simulink library "libraries"  (R2016b)
settings: Solver=VariableStepAuto  StartTime=0.0  StopTime=10.0  RelTol=1e-3
values from neighbouring files (symbols this model uses):
  MIN_SAFE_DIST = 1    [simulation.m]    (also in stateflowSim.m)
  WORLD_SIZE = 8    [simulation.m]    (also in stateflowSim.m)
undefined symbols (not defined in the file or in its folder): dt, V_MIN, V_TURN
settings Model: Creator=larry  LastModifiedBy=larry

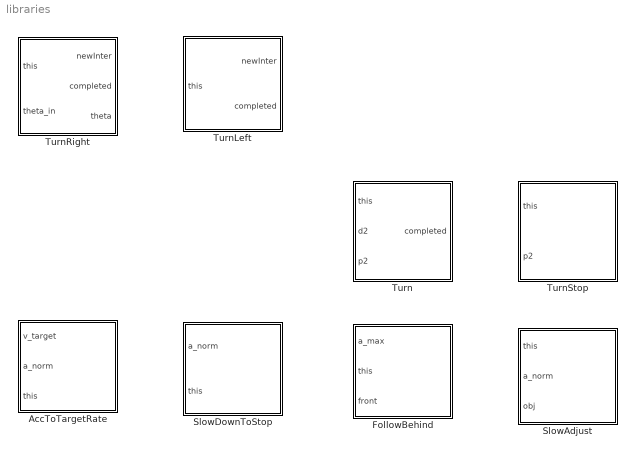
== system libraries ==
  AccToTargetRate : Stateflow chart  TreatAsAtomicUnit=on
  FollowBehind : Stateflow chart  TreatAsAtomicUnit=on
  SlowAdjust : Stateflow chart  TreatAsAtomicUnit=on
  SlowDownToStop : Stateflow chart  TreatAsAtomicUnit=on
  Turn : Stateflow chart  TreatAsAtomicUnit=on
  TurnLeft : Stateflow chart  TreatAsAtomicUnit=on
  TurnRight : Stateflow chart  TreatAsAtomicUnit=on
  TurnStop : Stateflow chart  TreatAsAtomicUnit=on

== stateflow chart libraries/AccToTargetRate ==
  state AccFromStop
    en:
    a = D(:,this) * a_norm;
    du:
    accelerate(this);
  state FixRate
    en:
    a = D(:,this) * 0;
    du:
    fixedRateDrive(this);
  (default) -> AccFromStop [order 2]
  AccFromStop -> FixRate : [reachTargetRate(this)]
  (default) -> FixRate [order 1] : [reachTargetRate(this)]
  data: self function_input uint8 size=1; self function_input uint8 size=1; self function_input uint8 size=1; res function_output boolean size=1; V data_store_memory; D data_store_memory; v_target input double size=1; a_norm input double size=1; this input uint8 size=1 =uint8(1); WORLD_SIZE parameter; a local double size=[2 1]; dt parameter; X data_store_memory
  function fixedRateDrive(self):
    | function fixedRateDrive(self)
    |  
    | x = X(:,self);
    | v = V(:,self);
    | 
    | % update new position
    | x = x + v * dt;
    | 
    | % a rounded world
    | if x(1) > WORLD_SIZE
    |     x(1) = -WORLD_SIZE;
    | elseif x(1) < -WORLD_SIZE
    |     x(1) = WORLD_SIZE;
    | elseif x(2) > WORLD_SIZE
    |     x(2) = -WORLD_SIZE;
    | elseif x(2) < -WORLD_SIZE
    |     x(2) = WORLD_SIZE;
    | end
    | 
    | X(:,self) = x;
  function accelerate(self):
    | function accelerate(self)
    | 
    | x = X(:,self);
    | v = V(:,self);
    | 
    | x = x + v * dt + 0.5 * a * dt * dt;
    | v = v + a * dt;
    | 
    | % a rounded world
    | if x(1) > WORLD_SIZE
    |     x(1) = -WORLD_SIZE;
    | elseif x(1) < -WORLD_SIZE
    |     x(1) = WORLD_SIZE;
    | elseif x(2) > WORLD_SIZE
    |     x(2) = -WORLD_SIZE;
    | elseif x(2) < -WORLD_SIZE
    |     x(2) = WORLD_SIZE;
    | end
    | 
    | X(:,self) = x;
    | V(:,self) = v;
  function res = reachTargetRate(self):
    | function res = reachTargetRate(self)
    | 
    | res = (norm(V(:,self)) >= v_target);

== stateflow chart libraries/SlowDownToStop ==
  state SlowToStop
    en:
    a = (-1) * D(:,this) * a_norm;
    du:
    accelerate(this);
  state Stop
    en:
    a = D(:,this) * 0;
    V(:,this) = V(:,this) * 0;
  (default) -> SlowToStop [order 2]
  SlowToStop -> Stop : [isStopped(this)]
  (default) -> Stop [order 1] : [isStopped(this)]
  data: self function_input uint8 size=1; self function_input uint8 size=1; res function_output boolean size=1; V data_store_memory; D data_store_memory; a_norm input double size=1; this input uint8 size=1 =uint8(1); WORLD_SIZE parameter; a local double size=[2 1]; dt parameter; X data_store_memory; V_MIN parameter
  function accelerate(self):
    | function accelerate(self)
    | 
    | x = X(:,self);
    | v = V(:,self);
    | 
    | x = x + v * dt + 0.5 * a * dt * dt;
    | v = v + a * dt;
    | 
    | % a rounded world
    | if x(1) > WORLD_SIZE
    |     x(1) = -WORLD_SIZE;
    | elseif x(1) < -WORLD_SIZE
    |     x(1) = WORLD_SIZE;
    | elseif x(2) > WORLD_SIZE
    |     x(2) = -WORLD_SIZE;
    | elseif x(2) < -WORLD_SIZE
    |     x(2) = WORLD_SIZE;
    | end
    | 
    | X(:,self) = x;
    | V(:,self) = v;
  function res = isStopped(self):
    | function res = isStopped(self)
    | 
    | v = V(:,self);
    | d = D(:,self);
    | res = (dot(v, d) <= 0)||(norm(v) < V_MIN);

== stateflow chart libraries/FollowBehind ==
  state Follow
    du:
    followFrontCar(this,front)
  (default) -> Follow
  data: self function_input uint8 size=1; index function_input uint8 size=1; V data_store_memory; D data_store_memory; a_max input double size=1; this input uint8 size=1 =uint8(1); WORLD_SIZE parameter; dt parameter; X data_store_memory; front input; MIN_SAFE_DIST parameter
  function followFrontCar(self, index):
    | function followFrontCar(self, index)
    | 
    | x = X(:,self);
    | v = V(:,self);
    | d = D(:,self);
    | a = [0; 0];
    | 
    | xfront = X(:,index);
    | vfront = V(:,index);
    | 
    | range = 2 * WORLD_SIZE;
    | dist = mod((dot(xfront - x, d)+range), range);
    | 
    | v_norm = norm(v);
    | vfront_norm = dot(vfront, d);
    | 
    | if dist <= 2*MIN_SAFE_DIST 
    |     
    |     if v_norm >= vfront_norm 
    |         vo = d * vfront_norm;
    |         if dist <= 1.5*MIN_SAFE_DIST
    |             vo = 0.75*vo;
    |         elseif dist <= MIN_SAFE_DIST
    |             vo = 0.5*vo;
    |         end
    |     else
    |         if dist <= MIN_SAFE_DIST
    |             vo = d * (v_norm + (vfront_norm - v_norm)*0.2);
    |         else
    |             vo = d * (v_norm + (vfront_norm - v_norm)*0.4);
    |         end
    |     end
    |     
    |     ar = (vo - v) / dt;
    |     ar_norm = norm(ar);
    |     if ar_norm > a_max
    |         ar = ar/ar_norm * a_max;
    |         x = x + v * dt + 0.5 * ar * dt * dt;
    |         v = v + ar * dt;
    |     else
    |         x = x + (v + vo) * dt / 2;
    |         v = vo;
    |     end
    |     a = ar;
    | else
    |     x = x + v * dt;
    | end
    | 
    | % a rounded world
    | if x(1) > WORLD_SIZE
    |     x(1) = -WORLD_SIZE;
    | elseif x(1) < -WORLD_SIZE
    |     x(1) = WORLD_SIZE;
    | elseif x(2) > WORLD_SIZE
    |     x(2) = -WORLD_SIZE;
    | elseif x(2) < -WORLD_SIZE
    |     x(2) = WORLD_SIZE;
    | end
    | 
    | X(:,self) = x;
    | V(:,self) = v;

== stateflow chart libraries/SlowAdjust ==
  state SlowDown
    en:
    a = (-1) * D(:,this) * a_norm;
    du:
    accelerate(this);
  state Adjust
    du:
    adjustBehind(this,obj)
  (default) -> SlowDown [order 2]
  SlowDown -> Adjust : [isStopped(this)]
  (default) -> Adjust [order 1] : [isStopped(this)]
  data: self function_input uint8 size=1; self function_input uint8 size=1; res function_output boolean size=1; self function_input uint8 size=1; pos function_input double size=[2 1]; V data_store_memory; D data_store_memory; this input uint8 size=1 =uint8(1); WORLD_SIZE parameter; dt parameter; X data_store_memory; MIN_SAFE_DIST parameter; V_MIN parameter; a local; a_norm input double size=1; obj input double size=[2 1]
  function accelerate(self):
    | function accelerate(self)
    | 
    | x = X(:,self);
    | v = V(:,self);
    | 
    | x = x + v * dt + 0.5 * a * dt * dt;
    | v = v + a * dt;
    | 
    | % a rounded world
    | if x(1) > WORLD_SIZE
    |     x(1) = -WORLD_SIZE;
    | elseif x(1) < -WORLD_SIZE
    |     x(1) = WORLD_SIZE;
    | elseif x(2) > WORLD_SIZE
    |     x(2) = -WORLD_SIZE;
    | elseif x(2) < -WORLD_SIZE
    |     x(2) = WORLD_SIZE;
    | end
    | 
    | X(:,self) = x;
    | V(:,self) = v;
  function res = isStopped(self):
    | function res = isStopped(self)
    | 
    | v = V(:,self);
    | d = D(:,self);
    | res = (dot(v, d) <= 0)||(norm(v) < V_MIN);
  function adjustBehind(self,pos):
    | function adjustBehind(self,pos)
    | 
    | x = X(:,self);
    | v = V(:,self);
    | d = D(:,self);
    | 
    | assert(norm(v) <= V_MIN);
    | 
    | diff = dot(pos - x, d);
    | if diff > MIN_SAFE_DIST
    |     v = V_MIN * d;
    |     dx_norm = V_MIN * dt;
    |     if (diff - dx_norm) >= MIN_SAFE_DIST
    |         x = x + dx_norm * d;
    |     else
    |         x = pos - MIN_SAFE_DIST * d;
    |     end
    | else
    |     v = 0 * v;
    | end
    | 
    | X(:,self) = x;
    | V(:,self) = v;

== stateflow chart libraries/TurnRight ==
  state Turn
    en:
    prepareRightTurn(this);
    check = false;
    du:
    check = rightTurn(this);
  state Resume
    en:
    newInter = ...
    resumeFromRightTurn(this);
    completed = true;
  (default) -> Turn
  Turn -> Resume : [check]
  data: self function_input uint8 size=1; self function_input uint8 size=1; res function_output boolean size=1; self function_input uint8 size=1; inter function_output double size=[2 1]; V data_store_memory; D data_store_memory; this input uint8 size=1 =uint8(1); dt parameter; X data_store_memory; dth local double size=1 =10; p0 local; x0 local; d0 local; newInter output; check local; completed output; vturn local; theta_in input; theta output double size=1 =0
  function prepareRightTurn(self):
    | function prepareRightTurn(self)
    | 
    | r = 0.5;
    | d0 = D(:,self);
    | theta = theta_in;
    | vturn = r * deg2rad(dth) / dt;
    | 
    | if isequal(d0, [1; 0])
    |     x0 = [-1; -0.5];
    |     p0 = [0; 0.5];
    | elseif isequal(d0, [-1; 0])
    |     x0 = [1; 0.5];
    |     p0 = [0; -0.5];
    | elseif isequal(d0, [0; 1])
    |     x0 = [0.5; -1];
    |     p0 = [-0.5; 0];
    | elseif isequal(d0, [0; -1])
    |     x0 = [-0.5; 1];
    |     p0 = [0.5; 0];
    | else
    |     error('Unknown orientation');
    | end
  function res = rightTurn(self):
    | function res = rightTurn(self)
    | 
    | res = false;
    | theta = theta + dth;
    | rad = deg2rad(theta);
    | 
    | rot = [cos(rad) sin(rad); -sin(rad) cos(rad)];
    | pf = rot * p0;
    | df = rot * d0;
    | 
    | diff = pf - p0;
    | 
    | % update states
    | X(:,self) = x0 + diff;
    | V(:,self) = df * vturn;
    | D(:,self) = df;
    | 
    | res = theta >= 90;
  function inter = resumeFromRightTurn(self):
    | function inter = resumeFromRightTurn(self)
    | 
    | if isequal(d0, [1; 0])
    |     df = [0; -1];
    |     xf = [-0.5; -1];
    |     inter = [-0.5; 1];
    | elseif isequal(d0, [-1; 0])
    |     df = [0; 1];
    |     xf = [0.5; 1];
    |     inter = [-0.5; -1];
    | elseif isequal(d0, [0; 1])
    |     df = [1; 0];
    |     xf = [1; -0.5];
    |     inter = [-1; -0.5];
    | elseif isequal(d0, [0; -1])
    |     df = [-1; 0];
    |     xf = [-1; 0.5];
    |     inter = [1; 0.5];
    | else
    |     error('Unknown orientation');
    | end
    | 
    | X(:,self) = xf;
    | V(:,self) = df * vturn;
    | D(:,self) = df;

== stateflow chart libraries/TurnLeft ==
  state Turn
    en:
    prepareLeftTurn(this);
    check = false;
    du:
    check = leftTurn(this);
  state Resume
    en:
    newInter = ...
    resumeFromLeftTurn(this);
    completed = true;
  (default) -> Turn
  Turn -> Resume : [check]
  data: self function_input uint8 size=1; self function_input uint8 size=1; res function_output boolean size=1; self function_input uint8 size=1; inter function_output double size=[2 1]; V data_store_memory; D data_store_memory; this input uint8 size=1 =uint8(1); dt parameter; X data_store_memory; dth local double size=1 =3.3; theta local; p0 local; x0 local; d0 local; newInter output; check local; completed output; vturn local
  function prepareLeftTurn(self):
    | function prepareLeftTurn(self)
    | 
    | r = 1.5;
    | d0 = D(:,self);
    | theta = 0;
    | vturn = r * deg2rad(dth) / dt;
    | 
    | if isequal(d0, [1; 0])
    |     x0 = [-1; -0.5];
    |     p0 = [0; -1.5];
    | elseif isequal(d0, [-1; 0])
    |     x0 = [1; 0.5];
    |     p0 = [0; 1.5];
    | elseif isequal(d0, [0; 1])
    |     x0 = [0.5; -1];
    |     p0 = [1.5; 0];
    | elseif isequal(d0, [0; -1])
    |     x0 = [-0.5; 1];
    |     p0 = [-1.5; 0];
    | else
    |     error('Unknown orientation');
    | end
  function res = leftTurn(self):
    | function res = leftTurn(self)
    | 
    | res = false;
    | theta = theta + dth;
    | rad = deg2rad(theta);
    | 
    | if theta > 90
    |     res = true;
    |     return;
    | end
    | 
    | rot = [cos(rad) -sin(rad); sin(rad) cos(rad)];
    | pf = rot * p0;
    | df = rot * d0;
    | 
    | diff = pf - p0;
    | 
    | X(:,self) = x0 + diff;
    | V(:,self) = df * vturn;
    | D(:,self) = df;
  function inter = resumeFromLeftTurn(self):
    | function inter = resumeFromLeftTurn(self)
    | 
    | if isequal(d0, [1; 0])
    |     df = [0; 1];
    |     xf = [0.5; 1];
    |     inter = [0.5; -1];
    | elseif isequal(d0, [-1; 0])
    |     df = [0; -1];
    |     xf = [-0.5; -1];
    |     inter = [-0.5; 1];
    | elseif isequal(d0, [0; 1])
    |     df = [-1; 0];
    |     xf = [-1; 0.5];
    |     inter = [1; 0.5];
    | elseif isequal(d0, [0; -1])
    |     df = [1; 0];
    |     xf = [1; -0.5];
    |     inter = [-1; -0.5];
    | else
    |     error('Unknown orientation');
    | end
    | 
    | X(:,self) = xf;
    | V(:,self) = df * vturn;
    | D(:,self) = df;

== stateflow chart libraries/Turn ==
  state Turn
    en:
    computeBezier2(this,p2,d2);
    check = false;
    du:
    completed = turnDrive(this);
  (default) -> Turn
  data: self function_input uint8 size=1; pf function_input double size=[2 1]; df function_input double size=[2 1]; self function_input uint8 size=1; res function_output boolean size=1; res function_output double size=1; pi function_input double size=[2 1]; pm function_input double size=[2 1]; pf function_input double size=[2 1]; V data_store_memory; D data_store_memory; this input uint8 size=1 =uint8(1); dt parameter; X data_store_memory; dth local double size=1 =1; p0 local; p1 local; completed output; d2 input; p2 input; check local; th local double size=1 =0; V_TURN parameter
  function computeBezier2(self, pf, df):
    | function computeBezier2(self, pf, df)
    | 
    | p0 = X(:,self);
    | d0 = D(:,self);
    | th = 0;
    | 
    | % p2 and d2 should be derived by high level calculation
    | [res, p1] = intersection(p0, d0, pf, df);
    | 
    | % model the time required to finish turns
    | dth = dthComputation(p0, p1, pf);
    | % dth = 0.1;
    | 
    | assert(res);
    | 
    | 
    | function [res, p_mid] = intersection(pi, di, pf, df)
    | 
    | xi = pi(1);
    | yi = pi(2);
    | ai = di(1);
    | bi = di(2);
    | xf = pf(1);
    | yf = pf(2);
    | af = df(1);
    | bf = df(2);
    | 
    | assert(norm(di) ~= 0 && norm(df) ~= 0);
    | 
    | 
    | p_mid = pi;
    | 
    | dp = pf - pi;
    | dp_norm = norm(dp);
    | if dp_norm == 0
    |     res = true;
    |     p_mid = pi;
    |     disp('pi and pf are overlapped');
    |     return;
    | end
    | 
    | dp = dp/dp_norm;
    | if bi == 0
    |     if bf == 0
    |         if isequal(dp, [ai/abs(ai); 0])
    |             res = true;
    |             p_mid = pf;
    |         else
    |             res = false;
    |         end
    |     else
    |         tf = (yi - yf)/bf;
    |         res = true;
    |         p_mid = [xf + af*tf; yf + bf*tf];
    |     end
    | else
    |     denominator = af*bi - ai*bf;
    |     if denominator == 0
    |         % parallel vector
    |         di = di/norm(di);
    |         if isequal(dp, di)
    |             res = true;
    |             p_mid = pf;
    |         else
    |             res = false;
    |         end
    |     else
    |         tf = ((bi*xi-ai*yi) - (bi*xf - ai*yf))/denominator;
    |         res = true;
    |         p_mid = [xf + af*tf; yf + bf*tf];
    |     end
    | end
  function res = turnDrive(self):
    | function res = turnDrive(self)
    | 
    | res = false;
    | x = X(:,self);
    | 
    | th = th + dth;
    | if th > 1
    |     res = true;
    |     return;
    | end
    | 
    | q0 = p0 * (1-th) + p1 * th;
    | q1 = p1 * (1-th) + p2 * th;
    | 
    | v = q1 - q0;
    | v = v/norm(v);
    | 
    | D(:,self) = v;
    | 
    | p = (1 - 2*th + th*th) * p0 + (2*th - 2*th*th) * p1 + (th*th)* p2;
    | dx = p - x;
    | v = v*norm(dx)/dt;
    | 
    | X(:,self) = p;
    | V(:,self) = v;
  function res = dthComputation(pi, pm, pf):
    | function res = dthComputation(pi, pm, pf)
    | 
    | last = pi;
    | length = 0;
    | for i=0:0.01:1
    |     p = (1 - 2*i + i*i) * pi + (2*i - 2*i*i) * pm + (i*i)* pf;
    |     length = length + norm(p - last);
    |     last = p;
    | end
    | res = dt*V_TURN/length;

== stateflow chart libraries/TurnStop ==
  state TurnStop
    en:
    V(:,this) = [0; 0];
  (default) -> TurnStop
  data: self function_input uint8 size=1; pf function_input double size=[2 1]; df function_input double size=[2 1]; self function_input uint8 size=1; res function_output boolean size=1; V data_store_memory; D data_store_memory; this input uint8 size=1 =uint8(1); dt parameter; X data_store_memory; dth local double size=1 =10; p0 local; p1 local; p2 input; th local double size=1 =0
  function computeBezier2(self, pf, df):
    | function computeBezier2(self, pf, df)
    | 
    | p0 = X(:,self);
    | d0 = D(:,self);
    | th = 0;
    | dth = 0.1;
    | 
    | % p2 and d2 should be derived by high level calculation
    | [res, p1] = intersection(p0, d0, pf, df);
    | 
    | assert(res);
    | 
    | 
    | function [res, p_mid] = intersection(pi, di, pf, df)
    | 
    | xi = pi(1);
    | yi = pi(2);
    | ai = di(1);
    | bi = di(2);
    | xf = pf(1);
    | yf = pf(2);
    | af = df(1);
    | bf = df(2);
    | 
    | assert(norm(di) ~= 0 && norm(df) ~= 0);
    | 
    | 
    | p_mid = pi;
    | 
    | dp = pf - pi;
    | dp_norm = norm(dp);
    | if dp_norm == 0
    |     res = true;
    |     p_mid = pi;
    |     disp('pi and pf are overlapped');
    |     return;
    | end
    | 
    | dp = dp/dp_norm;
    | if bi == 0
    |     if bf == 0
    |         if isequal(dp, [ai/abs(ai); 0])
    |             res = true;
    |             p_mid = pf;
    |         else
    |             res = false;
    |         end
    |     else
    |         tf = (yi - yf)/bf;
    |         res = true;
    |         p_mid = [xf + af*tf; yf + bf*tf];
    |     end
    | else
    |     denominator = af*bi - ai*bf;
    |     if denominator == 0
    |         % parallel vector
    |         di = di/norm(di);
    |         if isequal(dp, di)
    |             res = true;
    |             p_mid = pf;
    |         else
    |             res = false;
    |         end
    |     else
    |         tf = ((bi*xi-ai*yi) - (bi*xf - ai*yf))/denominator;
    |         res = true;
    |         p_mid = [xf + af*tf; yf + bf*tf];
    |     end
    | end
  function res = turnAccDrive(self):
    | function res = turnAccDrive(self)
    | 
    | res = false;
    | x = X(:,self);
    | 
    | th = th + dth;
    | if th > 1
    |     res = true;
    |     return;
    | end
    | 
    | q0 = p0 * (1-th) + p1 * th;
    | q1 = p1 * (1-th) + p2 * th;
    | 
    | v = q1 - q0;
    | v = v/norm(v);
    | 
    | D(:,self) = v;
    | 
    | p = (1 - 2*th + th*th) * p0 + (2*th - 2*th*th) * p1 + (th*th)* p2;
    | dx = p - x;
    | v = v*norm(dx)/dt;
    | 
    | X(:,self) = p;
    | V(:,self) = v;
